simulink model "dc_motor"  (R2025a)
settings: Solver=VariableStepAuto  StartTime=0.0  StopTime=10.0  RelTol=1e-3
settings Model: Creator=user  LastModifiedBy=user

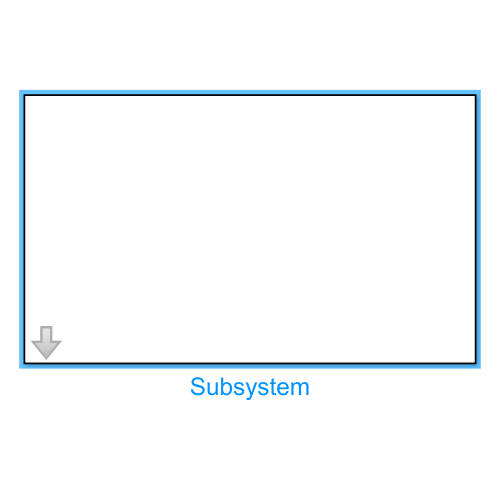
[thumbnail: Simulink's stored preview of the top-level diagram]
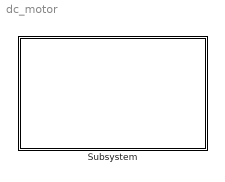
== system dc_motor ==
  Subsystem : Subsystem  mask{R_anchor=8, C_m=1.3, C_w=3.15, J_motor=0.000007, L_anchor=0.0015, L_ov=0.013, b=0.001}
      mask prompts: R_anchor "8"; C_m "1.3"; C_w "3.15"; J_motor "0.000007"; L_anchor "0.0015"; L_ov "0.013"; b "0.001"

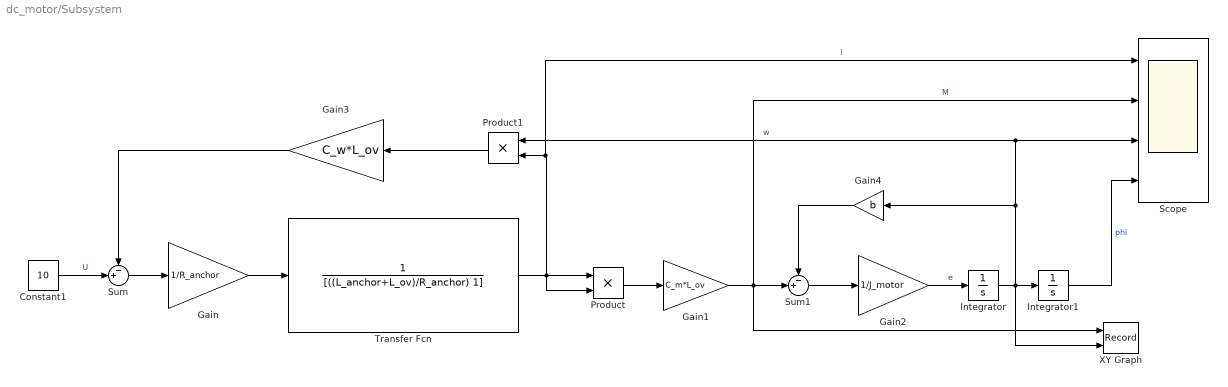
== system dc_motor/Subsystem ==
  Constant1 : Constant  Value=10
  Gain : Gain  Gain=1/R_anchor
  Gain1 : Gain  Gain=C_m*L_ov
  Gain2 : Gain  Gain=1/J_motor
  Gain3 : Gain  Gain=C_w*L_ov
  Gain4 : Gain  Gain=b
  Integrator : Integrator
  Integrator1 : Integrator
  Product : Product
  Product1 : Product
  Scope : Scope  NumInputPorts=4
      settings: ActiveDisplayString=4  ActiveDisplayYMinimum=-1236.7482389583179  ActiveDisplayYMaximum=11130.734150624863
  Sum : Sum  Inputs=-+|
  Sum1 : Sum  Inputs=-+|
  Transfer Fcn : TransferFcn  Denominator=[((L_anchor+L_ov)/R_anchor) 1]
  XY Graph : Record  NumPorts=2.0  FileSettingsInternal="{\"entries\":[{\"content\":{\"excelSettings\":{\"content\":{},\"type\":\"Streamout.ExcelSettings\"},\"parquetSettings\":{\"content\":{},\"type\":\"Streamout.ParquetSettings\"}},\"type\":\"Streamout.FileSettingStorage\",\"uuid\":\"\"}],\"packageUris\":[\"http:\\/\\/schema.mathworks.com\\/mf0\\/streamout_blocks\\/R2020a\"],\"version\":\"1.0\"}"  FrameSettings=[0, 0]  Layout=[1 1]  SignalsInternal="{\"entries\":[{\"content\":{\"signals\":[{\"content\":{\"blockPath\":[],\"dimensions\":[1],\"domain\":\"\",\"lineColor\":\"#a2142f\",\"plots\":[ 1 ],\"port\":1,\"sid\":[\"\"],\"signalID\":1,\"signalName\":\"M\"},\"type\":\"RecordBlkView.Signal\",\"uuid\":\"\"},{\"content\":{\"blockPath\":[],\"dimensions\":[1],\"domain\":\"\",\"lineColor\":\"#139fff\",\"plots\":[ 1 ],\"port\":2,\"sid\":[\"\"],\"signalID\":2,\"signalName\":\"w\"},\"type\":\"RecordBlkView.Signal\",\"uuid\":\"\"}]},\"type\":\"RecordBlkView.InputSignals\",\"uuid\":\"\"}],\"packageUris\":[\"http:\\/\\/schema.mathworks.com\\/mf0\\/streamout_blocks\\/R2020a\"],\"version\":\"1.0\"}"  VisualizationBindings="{\"xyplotplugin\":{\"info\":[{\"series\":[{\"bindingParametersList\":[{\"parameter\":\"X-Axis\",\"signalID\":1,\"signalName\":\"M\"},{\"parameter\":\"Y-Axis\",\"signalID\":2,\"signalName\":\"w\"}],\"seriesID\":0}],\"subplotID\":1}]}}"  CompatibilityTag=XY
  wires:
  Sum/1 -> Gain/1
  Constant1/1 -> Sum/2  "U"
  Gain/1 -> Transfer Fcn/1
  Transfer Fcn/1 -> Product/2, Product/1, Scope/1, Product1/2  "i"
  Product/1 -> Gain1/1
  Gain1/1 -> XY Graph/1, Scope/2, Sum1/2  "M"
  Gain4/1 -> Sum1/1
  Sum1/1 -> Gain2/1
  Gain2/1 -> Integrator/1  "e"
  Integrator/1 -> XY Graph/2, Gain4/1, Scope/3, Product1/1, Integrator1/1  "w"
  Integrator1/1 -> Scope/4  "phi"
  Product1/1 -> Gain3/1
  Gain3/1 -> Sum/1
